simulink model "Sim_OpenLoop"  (Simulink 10.0)
settings: Solver=VariableStepAuto  StartTime=0.0  StopTime=120  RelTol=1e-3
values from neighbouring files (symbols this model uses):
  Ac = pi*Dc^2/4    (= 0.00155179165474)    [Script_OpenLoop.m]
  Ao = pi*Do^2/4    (= 1.7813934812e-05)    [Script_OpenLoop.m]
  Cd = 0.9    [Script_OpenLoop.m]
  g = 9.81    [Script_OpenLoop.m]
  h0 = 0.1696    [Script_OpenLoop.m]
  Kp = ((Cd * Ao)./(pump_voltage - v_min)).*sqrt(2*g*height_ss)    [Script_OpenLoop.m]
  vp = 0    [Script_OpenLoop.m]
settings Model: Creator=jpk170130  LastModifiedBy=ancar
settings DataIOCC: SaveFormat=Dataset
settings OptimizationCC: LifeSpan=auto
settings DebuggingCC: UnderspecifiedInitializationDetection=Simplified  MergeDetectMultiDrivingBlocksExec=error  SFUnexpectedBacktrackingDiag=error  SFNoUnconditionalDefaultTransitionDiag=error  SFExecutionAtInitializationDiag=warning
settings HardwareCC: ProdBitPerPointer=64  ProdBitPerSizeT=64  ProdBitPerPtrDiffT=64  ProdLargestAtomicFloat=Float  ProdIntDivRoundTo=Zero  ProdEndianess=LittleEndian  ProdWordSize=64  ProdHWDeviceType=Intel->x86-64 (Windows64)
settings ModelReferenceCC: PropagateSignalLabelsOutOfModel=on
settings CodeAppCC: StateflowObjectComments=off
settings GRTTargetCC: TargetLangStandard=C99 (ISO)  CombineOutputUpdateFcns=on  GRTInterface=off
settings ConfigComp: CovMetricSettings=dwe  CovHtmlReporting=off  CovSaveCumulativeToWorkspaceVar=off  CovSaveSingleToWorkspaceVar=off

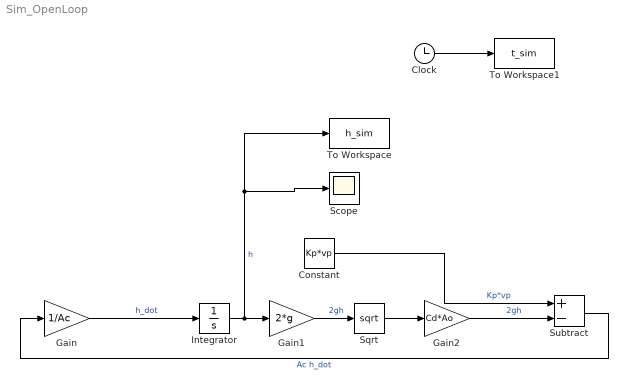
== system Sim_OpenLoop ==
  Clock : Clock
  Constant : Constant  Value=Kp*vp
  Gain : Gain  Gain=1/Ac
  Gain1 : Gain  Gain=2*g
  Gain2 : Gain  Gain=Cd*Ao
  Integrator : Integrator  InitialCondition=h0
  Scope : Scope
  Sqrt : Sqrt  SaturateOnIntegerOverflow=on
  Subtract : Sum  Inputs=+-
  To Workspace : ToWorkspace  VariableName=h_sim  SampleTime=0.1
  To Workspace1 : ToWorkspace  VariableName=t_sim  SampleTime=0.1
  wires:
  Integrator/1 -> Scope/1, To Workspace/1, Gain1/1  "h"
  Gain/1 -> Integrator/1  "h_dot"
  Constant/1 -> Subtract/1  "Kp*vp"
  Gain1/1 -> Sqrt/1  "2gh"
  Subtract/1 -> Gain/1  "Ac h_dot"
  Clock/1 -> To Workspace1/1
  Sqrt/1 -> Gain2/1
  Gain2/1 -> Subtract/2  "2gh"
